simulink model "S_ELECTRO_2025_MTET_NoInt_EnvDatos_V1"  (R2017a)
settings: Solver=FixedStepDiscrete  StartTime=0.0  StopTime=10.0  RelTol=1e-3
undefined symbols (not defined in the file or in its folder): Down, GPTRIP1SEL, GPTRIP2SEL, TZ1, TZ2, Up
libraries: c2802xlib x4, c2806xlib x2, simulink x1, c280xlib x1
settings Model: ExtModeTrigDuration=8  Creator=dricl  LastModifiedBy=dricl
settings OptimizationCC: DefaultUnderspecifiedDataType=single  PassReuseOutputArgsAs=Individual arguments  MaxStackSize=512
settings DebuggingCC: ParameterTunabilityLossMsg=error
settings HardwareCC: ProdBitPerChar=16  ProdBitPerInt=16  ProdBitPerPointer=32  ProdBitPerSizeT=32  ProdBitPerPtrDiffT=32  ProdLargestAtomicInteger=Integer  ProdLargestAtomicFloat=None  ProdWordSize=16  ProdLongLongMode=on  ProdHWDeviceType=Texas Instruments->C2000
settings SFSimCC: MATLABDynamicMemAlloc=off
settings RTWCC: SystemTargetFile=ert.tlc  HardwareBoard=TI Piccolo F2806x  TLCOptions=-aInlineSetEventsForThisBaseRateFcn=TLC_FALSE -aSuppressMultiTaskScheduler=TLC_FALSE -aRateBasedStepFcn=1  TemplateMakefile=ert_default_tmf  Description=Embedded Coder  Toolchain=Texas Instruments Code Composer Studio v5 (C2000)  CodeExecutionProfiling=on  CodeProfilingSaveOptions=AllData  CodeProfilingInstrumentation=on
settings CodeAppCC: ForceParamTrailComments=on  IgnoreCustomStorageClasses=off  OperatorAnnotations=on  SimulinkDataObjDesc=on  SFDataObjDesc=on  MATLABFcnDesc=on  InsertBlockDesc=on  MATLABSourceComments=on
settings ERTTargetCC: CodeReplacementLibrary=TI C28x  MemSecPackage=tic2000demospkg  MemSecFuncExecute=code_ramfuncs

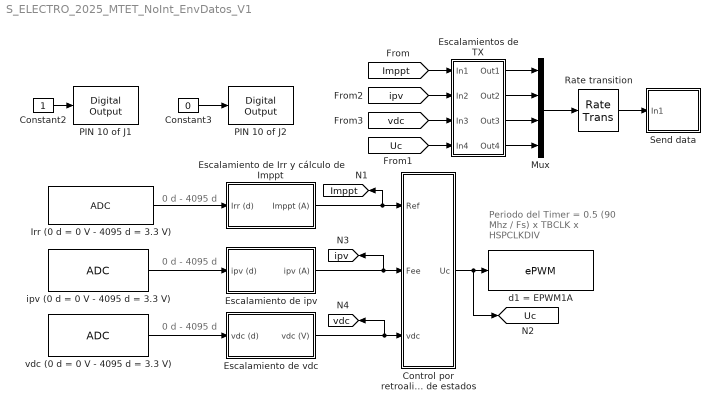
== system S_ELECTRO_2025_MTET_NoInt_EnvDatos_V1 ==
  note: 0 d - 4095 d
  note: Periodo del Timer =
      |  0.5 (90 Mhz / Fs)  x
      | TBCLK x HSPCLKDIV
  note: 0 d - 4095 d
  note: 0 d - 4095 d
  Constant2 : Constant  Priority=1  SampleTime=0.0002
  Constant3 : Constant  Priority=11  Value=0  SampleTime=0.0002
  Control por retroalimentación de estados : Subsystem  Priority=9  TreatAsAtomicUnit=on
  Escalamiento de Irr y cálculo de Imppt : Subsystem  Priority=6  TreatAsAtomicUnit=on
  Escalamiento de ipv : Subsystem  Priority=7  TreatAsAtomicUnit=on
  Escalamiento de vdc : Subsystem  Priority=8  TreatAsAtomicUnit=on
  Escalamientos de TX : Subsystem  TreatAsAtomicUnit=on
  "Irr (0 d = 0 V - 4095 d = 3.3 V) " : c2802xlib/ADC  Priority=3  ADCModule=1  samplingMode=Single sample mode  ADCResolution=12-bit (Single-ended input)  useSOC1=SOC1  useSOC2=SOC0_SOC1  SOCAcquisitionWindow=7  SOCTriggerSource=ePWM1_ADCSOCA  SOCInterruptTrigger=No ADCINT  Ts=0.0002  dType=uint16  postInterrupt=off  interruptSel=ADCINT1  ADCINTContinuous=on  endma=off  chdma=1  blkParamProc=C2000  conv1=ADCINA1  conv2=ADCINA0 and ADCINB0  conv1_Type4=ADCIN0  conv2_Type4=ADCIN0 and ADCIN1
      settings: SourceProductName=Embedded Coder Support Package for Texas Instruments C2000 Processors
  Mux : Mux
  PIN 10 of J1 : c2806xlib/Digital Output  Priority=2  GPIO_Number=GPIO32~GPIO39  GPIO_Bit0=on  GPIO_BIT0_Toggle=off  GPIO_Bit1=off  GPIO_BIT1_Toggle=off  GPIO_Bit2=off  GPIO_BIT2_Toggle=off  GPIO_Bit3=off  GPIO_BIT3_Toggle=off  GPIO_Bit4=off  GPIO_BIT4_Toggle=off  GPIO_Bit5=off  GPIO_BIT5_Toggle=off  GPIO_Bit6=off  GPIO_BIT6_Toggle=off  GPIO_Bit7=off  GPIO_BIT7_Toggle=off
      settings: SourceProductName=Embedded Coder Support Package for Texas Instruments C2000 Processors  SourceProductBaseCode=TIC2000
  PIN 10 of J2 : c2806xlib/Digital Output  Priority=12  GPIO_Number=GPIO32~GPIO39  GPIO_Bit0=on  GPIO_BIT0_Toggle=off  GPIO_Bit1=off  GPIO_BIT1_Toggle=off  GPIO_Bit2=off  GPIO_BIT2_Toggle=off  GPIO_Bit3=off  GPIO_BIT3_Toggle=off  GPIO_Bit4=off  GPIO_BIT4_Toggle=off  GPIO_Bit5=off  GPIO_BIT5_Toggle=off  GPIO_Bit6=off  GPIO_BIT6_Toggle=off  GPIO_Bit7=off  GPIO_BIT7_Toggle=off
      settings: SourceProductName=Embedded Coder Support Package for Texas Instruments C2000 Processors  SourceProductBaseCode=TIC2000
  Rate transition : RateTransition  Integrity=off  Deterministic=off  OutPortSampleTime=0.0002
  Send data : Subsystem  TreatAsAtomicUnit=on
  d1 = EPWM1A : c2802xlib/ePWM  Priority=10  useModule=ePWM1  ePWMxLINKTBPRD=Not Linked  periodUnits=Clock cycles  timerSource=Specify via dialog  timerPeriod_clk=9000  timerPeriod_sec=0.0001  tbshadow=Counter equals to zero  countingMode=Up-Down  phaseActiveEnable=Disable  phaseDirection=Count down after sync  phaseActive=0  synchronizationEnable=off  dcaevt1Sync=off  dcbevt1Sync=off  synchronizationOption=Disable  clockPrescale=1  HSclockPrescale=1  enswap=off  ePWMxAStatus=on  ePWMxAactionLogic1=Do nothing  ePWMxAactionLogic2=Do nothing  ePWMxAactionLogic3=Clear  ePWMxAactionLogic4=Set  ePWMxAactionLogic5=Do nothing  ePWMxAactionLogic6=Do nothing  ePWMxALoadMode=Load on counter equals to zero (CTR=Zero)  ePWMxACSFenable=off  ePWMxACSFvalue=Forcing disable  ePWMxASFreload=Zero  ePWMxBStatus=off  ePWMxBactionLogic1=Set  ePWMxBactionLogic2=Clear  ePWMxBactionLogic3=Do nothing  ePWMxBactionLogic4=Do nothing  ePWMxBactionLogic5=Clear  ePWMxBactionLogic6=Set  ePWMxBLoadMode=Load on counter equals to zero (CTR=Zero)  ePWMxBCSFenable=off  ePWMxBCSFvalue=Forcing disable  ePWMxBSFreload=Zero  ePWNxBOutWay=off  ePWMxLINKCMPA=Not Linked  CMPAUnits=Clock cycles  CMPASource=Input port  CMPAValue_per=50  CMPAValue_clk=4500  enCMPAshadow=Counter equals to zero  ePWMxLINKCMPB=Not Linked  CMPBUnits=Clock cycles  CMPBSource=Specify via dialog  CMPBValue_per=50  CMPBValue_clk=4500  enCMPBshadow=Counter equals to zero  ePWMxLINKCMPC=Not Linked  CMPCUnits=Clock cycles  CMPCSource=Specify via dialog  CMPCValue_per=50  CMPCValue_clk=32000  enCMPCshadow=Counter equals to zero  ePWMxLINKCMPD=Not Linked  CMPDUnits=Clock cycles  CMPDSource=Specify via dialog  CMPDValue_per=50  CMPDValue_clk=32000  enCMPDshadow=Counter equals to zero  enableDBePWMxA=on  enableDBePWMxB=on  enhalfcycle=off  DBpolarity=Active high complementary (AHC)  DBedgeDelay=Positive  DBSource_ePWMxA=ePWMxA  DBSource_ePWMxB=ePWMxA  DBperiodSource=Specify via dialog  REDperiod=50  FEDperiod=50  adcstartModuleA=on  adcrequestEventA=First event  adcstartEventA=Counter equals to period (CTR=PRD)  adcstartEventA_type2=Digital Compare Module A Event 1 start of conversion (DCAEVT1.soc)  adcstartModuleB=off  adcrequestEventB=First event  adcstartEventB=Counter equals to zero (CTR=Zero)  adcstartEventB_type2=Counter equals to zero (CTR=Zero)  intEn=off  intPrd=First event  intSel=Counter equals to zero (CTR=Zero)  intSel_type2=Counter equals to zero (CTR=Zero)  hrpe=off  enHRPWM=off  HRPWM_LoadMode=Counter equals to period (CTR=PRD)  HRPWM_CTLMode=Duty or Period control mode  HRPWM_EDGMode=Both edge  hrpeb=off  enHRPWMB=off  HRPWM_LoadModeB=Counter equals to zero (CTR=ZERO)  HRPWM_CTLModeB=Duty or Period control mode  HRPWM_EDGModeB=Both edge  enSFO=on  enautoconv=on  chopperEnable=off  chopperFrequency=1  chopperFirstwidth=1  chopperDuty=12.5%  tripZonesource=Specify via dialog  tzselOSHT1=off  tzselOSHT2=off  tzselOSHT3=off  tzselOSHDCAEV1=off  tzselOSHDCBEV1=off  tzselCBC1=off  tzselCBC2=off  tzselCBC3=off  tzselCBCDCAEV2=off  tzselCBCDCBEV2=off  tzselOSHT4=off  tzselOSHT5=off  tzselOSHT6=off  tzselCBC4=off  tzselCBC5=off  tzselCBC6=off  enTzOstIntr=off  enTzCbcIntr=off  enTzDCAEVT1Intr=off  enTzDCAEVT2Intr=off  enTzDCBEVT1Intr=off  enTzDCBEVT2Intr=off  ePWMxAforced=No action  ePWMxBforced=No action  DCAEVT1forced=No action  DCBEVT1forced=No action  DCAEVT2forced=No action  DCBEVT2forced=No action  dcah=Trip Zone 1 input (TZ1)  dcal=Trip Zone 2 input (TZ2)  dcbh=Trip Zone 1 input (TZ1)  dcbl=Trip Zone 2 input (TZ2)  dcah_type2=GPTRIP1SEL/(TZ1)  dcal_type2=GPTRIP2SEL/(TZ2)  dcbh_type2=GPTRIP1SEL/(TZ1)  dcbl_type2=GPTRIP2SEL/(TZ2)  gendcaevt1=Event disabled  gendcaevt2=Event disabled  gendcbevt1=Event disabled  gendcbevt2=Event disabled  dcaevt1src=DCAEVT1 with sync  dcaevt2src=DCAEVT2 with sync  dcbevt1src=DCBEVT1 with sync  dcbevt2src=DCBEVT2 with sync  pulsesel=Counter equals to zero (CTR=Zero)  blankinv=off  blankoffset=0  blankwidth=0  evsrcsel=Filtered version of DCAEVT1 (DCAEVT1FILT)  encape=off  PwmType=C2000
      settings: SourceProductName=Embedded Coder Support Package for Texas Instruments C2000 Processors
  "ipv (0 d = 0 V - 4095 d = 3.3 V) " : c2802xlib/ADC  Priority=4  ADCModule=1  samplingMode=Single sample mode  ADCResolution=12-bit (Single-ended input)  useSOC1=SOC2  useSOC2=SOC0_SOC1  SOCAcquisitionWindow=7  SOCTriggerSource=ePWM1_ADCSOCA  SOCInterruptTrigger=No ADCINT  Ts=0.0002  dType=uint16  postInterrupt=off  interruptSel=ADCINT1  ADCINTContinuous=on  endma=off  chdma=1  blkParamProc=C2000  conv1=ADCINA0  conv2=ADCINA0 and ADCINB0  conv1_Type4=ADCIN0  conv2_Type4=ADCIN0 and ADCIN1
      settings: SourceProductName=Embedded Coder Support Package for Texas Instruments C2000 Processors
  "vdc (0 d = 0 V - 4095 d = 3.3 V) " : c2802xlib/ADC  Priority=5  ADCModule=1  samplingMode=Single sample mode  ADCResolution=12-bit (Single-ended input)  useSOC1=SOC3  useSOC2=SOC0_SOC1  SOCAcquisitionWindow=7  SOCTriggerSource=ePWM1_ADCSOCA  SOCInterruptTrigger=No ADCINT  Ts=0.0002  dType=uint16  postInterrupt=off  interruptSel=ADCINT1  ADCINTContinuous=on  endma=off  chdma=1  blkParamProc=C2000  conv1=ADCINA2  conv2=ADCINA0 and ADCINB0  conv1_Type4=ADCIN0  conv2_Type4=ADCIN0 and ADCIN1
      settings: SourceProductName=Embedded Coder Support Package for Texas Instruments C2000 Processors
  tag scope: Imppt=global, Uc=global, ipv=global, vdc=global
  wires:
  Escalamiento de ipv/1(ipv (A)) -> [ipv], Control por retroalimentación de estados/2(Fee)
  "ipv (0 d = 0 V - 4095 d = 3.3 V) "/1 -> Escalamiento de ipv/1(ipv (d))
  Escalamiento de Irr y cálculo de Imppt/1(Imppt (A)) -> [Imppt], Control por retroalimentación de estados/1(Ref)
  "Irr (0 d = 0 V - 4095 d = 3.3 V) "/1 -> Escalamiento de Irr y cálculo de Imppt/1(Irr (d))
  Constant2/1 -> PIN 10 of J1/1
  Constant3/1 -> PIN 10 of J2/1
  "vdc (0 d = 0 V - 4095 d = 3.3 V) "/1 -> Escalamiento de vdc/1(vdc (d))
  Escalamiento de vdc/1(vdc (V)) -> [vdc], Control por retroalimentación de estados/3(vdc)
  [vdc] -> Escalamientos de TX/3(In3)
  [ipv] -> Escalamientos de TX/2(In2)
  [Uc] -> Escalamientos de TX/4(In4)
  [Imppt] -> Escalamientos de TX/1(In1)
  Escalamientos de TX/2(Out2) -> Mux/2
  Escalamientos de TX/4(Out4) -> Mux/4
  Escalamientos de TX/3(Out3) -> Mux/3
  Escalamientos de TX/1(Out1) -> Mux/1
  Mux/1 -> Rate transition/1
  Rate transition/1 -> Send data/1(In1)
  Control por retroalimentación de estados/1(Uc) -> [Uc], d1 = EPWM1A/1

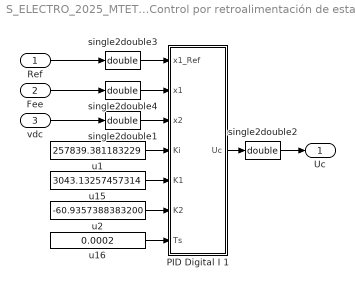
== system S_ELECTRO_2025_MTET_NoInt_EnvDatos_V1/Control por retroalimentación de estados ==
  Ref : Inport
  Fee : Inport  Port=2
  vdc : Inport  Port=3
  PID Digital I 1 : MATLAB Function  TreatAsAtomicUnit=on
  single2double{1..4} (4 alike) : DataTypeConversion  OutDataTypeStr=double
  u1 : Constant  Value=257839.381183229  SampleTime=0.0002
  u15 : Constant  Value=3043.13257457314  SampleTime=0.0002
  u16 : Constant  Value=0.0002  SampleTime=0.0002
  u2 : Constant  Value=-60.9357388383200  SampleTime=0.0002
  Uc : Outport
  wires:
  u16/1 -> PID Digital I 1/7(Ts)
  Ref/1 -> single2double3/1
  single2double2/1 -> Uc/1
  Fee/1 -> single2double4/1
  PID Digital I 1/1(Uc) -> single2double2/1
  single2double3/1 -> PID Digital I 1/1(x1_Ref)
  single2double4/1 -> PID Digital I 1/2(x1)
  u1/1 -> PID Digital I 1/4(Ki)
  vdc/1 -> single2double1/1
  single2double1/1 -> PID Digital I 1/3(x2)
  u15/1 -> PID Digital I 1/5(K1)
  u2/1 -> PID Digital I 1/6(K2)

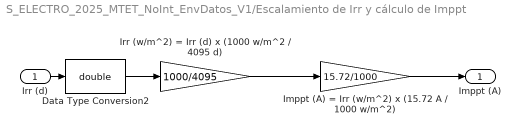
== system S_ELECTRO_2025_MTET_NoInt_EnvDatos_V1/Escalamiento de Irr y cálculo de Imppt ==
  Irr (d) : Inport
  Data Type Conversion2 : DataTypeConversion  OutDataTypeStr=double
  "Imppt (A) = Irr (w/m^2) x (15.72 A / 1000 w/m^2) " : Gain  Gain=15.72/1000
  Irr (w/m^2) = Irr (d) x (1000 w/m^2 / 4095 d) : Gain  Gain=1000/4095
  Imppt (A) : Outport
  wires:
  Irr (d)/1 -> Data Type Conversion2/1
  Data Type Conversion2/1 -> Irr (w/m^2) = Irr (d) x (1000 w/m^2 / 4095 d)/1
  Irr (w/m^2) = Irr (d) x (1000 w/m^2 / 4095 d)/1 -> "Imppt (A) = Irr (w/m^2) x (15.72 A / 1000 w/m^2) "/1
  "Imppt (A) = Irr (w/m^2) x (15.72 A / 1000 w/m^2) "/1 -> Imppt (A)/1

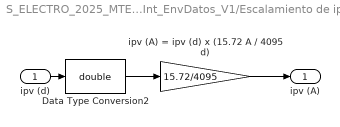
== system S_ELECTRO_2025_MTET_NoInt_EnvDatos_V1/Escalamiento de ipv ==
  ipv (d) : Inport
  Data Type Conversion2 : DataTypeConversion  OutDataTypeStr=double
  ipv (A) = ipv (d) x (15.72 A / 4095 d) : Gain  Gain=15.72/4095
  ipv (A) : Outport
  wires:
  ipv (d)/1 -> Data Type Conversion2/1
  Data Type Conversion2/1 -> ipv (A) = ipv (d) x (15.72 A / 4095 d)/1
  ipv (A) = ipv (d) x (15.72 A / 4095 d)/1 -> ipv (A)/1

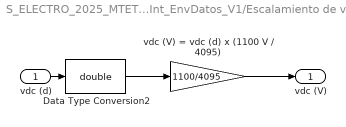
== system S_ELECTRO_2025_MTET_NoInt_EnvDatos_V1/Escalamiento de vdc ==
  vdc (d) : Inport
  Data Type Conversion2 : DataTypeConversion  OutDataTypeStr=double
  vdc (V) = vdc (d) x (1100 V / 4095) : Gain  Gain=1100/4095
  vdc (V) : Outport
  wires:
  Data Type Conversion2/1 -> vdc (V) = vdc (d) x (1100 V / 4095)/1
  vdc (d)/1 -> Data Type Conversion2/1
  vdc (V) = vdc (d) x (1100 V / 4095)/1 -> vdc (V)/1

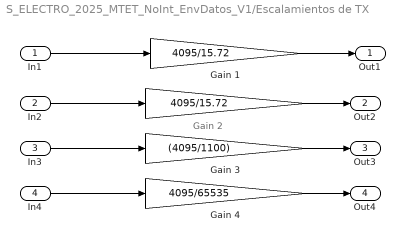
== system S_ELECTRO_2025_MTET_NoInt_EnvDatos_V1/Escalamientos de TX ==
  note: Gain 2
  In1 : Inport
  In2 : Inport  Port=2
  In3 : Inport  Port=3
  In4 : Inport  Port=4
  " " : Gain  Gain=4095/15.72  OutDataTypeStr=uint16  RndMeth=Simplest
  Gain 1 : Gain  Gain=4095/15.72  OutDataTypeStr=uint16  RndMeth=Simplest
  Gain 3 : Gain  Gain=(4095/1100)  OutDataTypeStr=uint16  RndMeth=Simplest
  Gain 4 : Gain  Gain=4095/65535  OutDataTypeStr=uint16  RndMeth=Simplest
  Out1 : Outport
  Out2 : Outport  Port=2
  Out3 : Outport  Port=3
  Out4 : Outport  Port=4
  wires:
  Gain 1/1 -> Out1/1
  " "/1 -> Out2/1
  Gain 3/1 -> Out3/1
  In1/1 -> Gain 1/1
  In2/1 -> " "/1
  In3/1 -> Gain 3/1
  In4/1 -> Gain 4/1
  Gain 4/1 -> Out4/1

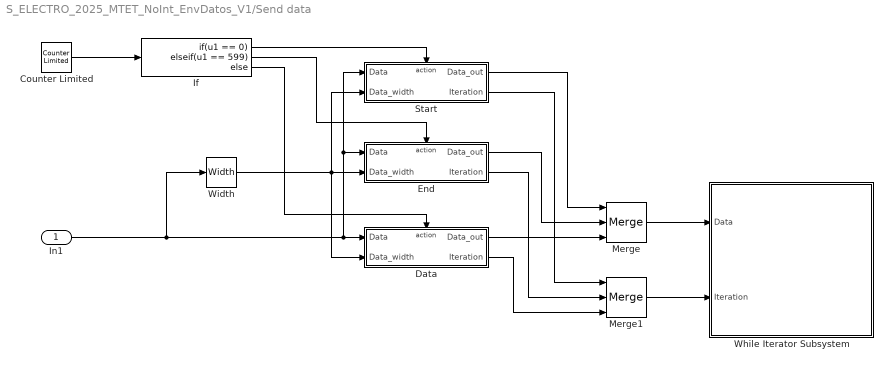
== system S_ELECTRO_2025_MTET_NoInt_EnvDatos_V1/Send data ==
  In1 : Inport
  Counter Limited : simulink/Sources/Counter Limited  uplimit=599  tsamp=-1
  Data : Subsystem  TreatAsAtomicUnit=on
  End : Subsystem  TreatAsAtomicUnit=on
  If : If  IfExpression=u1 == 0  ElseIfExpressions=u1 == 599
  Merge : Merge  Inputs=3
  Merge1 : Merge  Inputs=3
  Start : Subsystem  TreatAsAtomicUnit=on
  While Iterator Subsystem : Subsystem  TreatAsAtomicUnit=on
  Width : Width  OutDataTypeMode=All ports same datatype  DataType=uint16
  wires:
  If/1 -> Start/Action
  If/2 -> End/Action
  If/3 -> Data/Action
  Counter Limited/1 -> If/1
  Start/1(Data_out) -> Merge/1
  End/1(Data_out) -> Merge/2
  Data/1(Data_out) -> Merge/3
  Merge/1 -> While Iterator Subsystem/1(Data)
  Merge1/1 -> While Iterator Subsystem/2(Iteration)
  Start/2(Iteration) -> Merge1/1
  End/2(Iteration) -> Merge1/2
  Data/2(Iteration) -> Merge1/3
  In1/1 -> Width/1, Start/1(Data), End/1(Data), Data/1(Data)
  Width/1 -> Data/2(Data_width), Start/2(Data_width), End/2(Data_width)

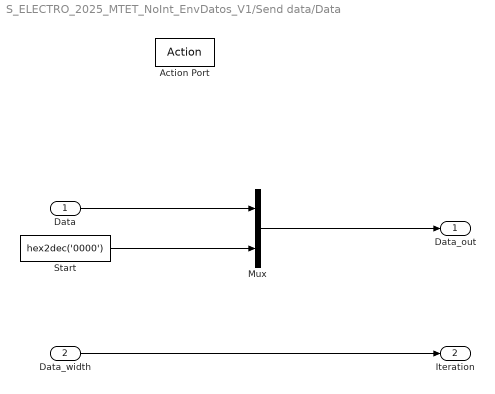
== system S_ELECTRO_2025_MTET_NoInt_EnvDatos_V1/Send data/Data ==
  Data : Inport
  Data_width : Inport  Port=2
  Action Port : ActionPort  ActionType=else
  Mux : Mux  Inputs=2
  Start : Constant  Value=hex2dec('0000')  OutDataTypeStr=uint16
  Data_out : Outport
  Iteration : Outport  Port=2
  wires:
  Start/1 -> Mux/2
  Mux/1 -> Data_out/1
  Data/1 -> Mux/1
  Data_width/1 -> Iteration/1

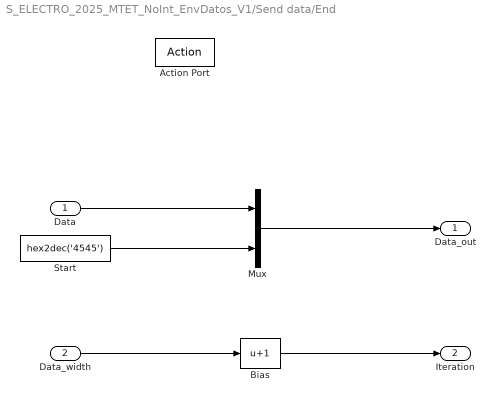
== system S_ELECTRO_2025_MTET_NoInt_EnvDatos_V1/Send data/End ==
  Data : Inport
  Data_width : Inport  Port=2
  Action Port : ActionPort  ActionType=elseif
  Bias : Bias  Bias=1
  Mux : Mux  Inputs=2
  Start : Constant  Value=hex2dec('4545')  OutDataTypeStr=uint16
  Data_out : Outport
  Iteration : Outport  Port=2
  wires:
  Mux/1 -> Data_out/1
  Data_width/1 -> Bias/1
  Start/1 -> Mux/2
  Bias/1 -> Iteration/1
  Data/1 -> Mux/1

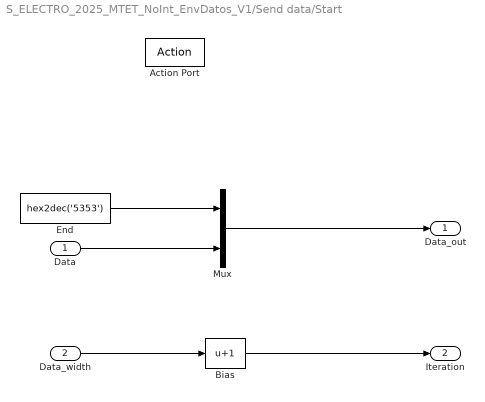
== system S_ELECTRO_2025_MTET_NoInt_EnvDatos_V1/Send data/Start ==
  Data : Inport
  Data_width : Inport  Port=2
  Action Port : ActionPort  ActionType=then
  Bias : Bias  Bias=1
  End : Constant  Value=hex2dec('5353')  OutDataTypeStr=uint16
  Mux : Mux  Inputs=2
  Data_out : Outport
  Iteration : Outport  Port=2
  wires:
  End/1 -> Mux/1
  Mux/1 -> Data_out/1
  Data_width/1 -> Bias/1
  Bias/1 -> Iteration/1
  Data/1 -> Mux/2

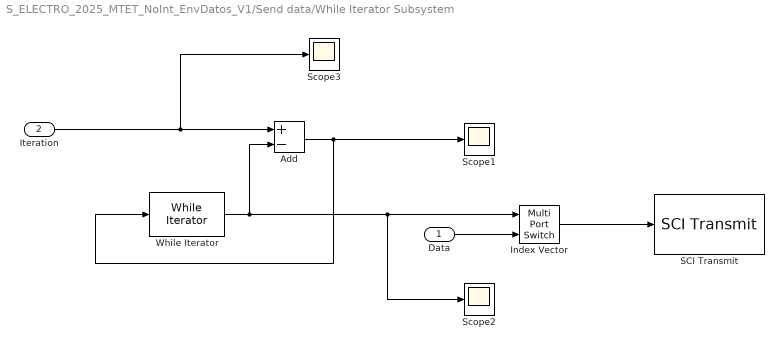
== system S_ELECTRO_2025_MTET_NoInt_EnvDatos_V1/Send data/While Iterator Subsystem ==
  Data : Inport
  Iteration : Inport  Port=2
  Add : Sum  Inputs=+-  OutDataTypeStr=Inherit: Same as first input
  Index Vector : MultiPortSwitch  Inputs=1
  SCI Transmit : c280xlib/SCI Transmit  sciModule=A  dataHead=''  dataTail=''  postInterrupt=off  numFifo=1
      settings: SourceProductName=Embedded Coder Support Package for Texas Instruments C2000 Processors
  Scope1 : Scope
  Scope2 : Scope
  Scope3 : Scope
  While Iterator : WhileIterator  MaxIters=-1  WhileBlockType=do-while  ShowIterationPort=on  OutputDataType=int16
  wires:
  Iteration/1 -> Scope3/1, Add/1
  Add/1 -> Scope1/1, While Iterator/1
  Index Vector/1 -> SCI Transmit/1
  Data/1 -> Index Vector/2
  While Iterator/1 -> Scope2/1, Index Vector/1, Add/2

== matlab function S_ELECTRO_2025_MTET_NoInt_EnvDatos_V1/Control por retroalimentación de estados/PID Digital I 1 ==
  data: x1_Ref input; x1 input; x2 input; Uc output; Ki input; K1 input; K2 input; Ts input
function Uc = fcn(x1_Ref, x1, x2, Ki, K1, K2, Ts)
    % Retroalimentación de estados con acción integral
    
    % Variables persistentes para mantener el estado entre llamadas
    persistent ek Acc_Int Acc_Int_1 uk
    
    if isempty(ek)
        ek = 0;
        Acc_Int = 0;
        Acc_Int_1 = 0;
        uk = 0;
    end

    % Cálculo del error
    ek = x1_Ref - x1;

    % Acción integral
    Acc_Int = Ki * ek * Ts + Acc_Int_1;
    Acc_Int_1 = Acc_Int;

    % Ley de control: acción integral menos retroalimentación de estados
    uk = Acc_Int - (K1 * x1 + K2 * x2);

    % Saturación (opcional)
    %uk = min(max(uk, 0), 65535); %Para med TET
     uk = min(max(uk, 0), 9000);  %Para pruebas de TX/RX 

    % Salida del controlador
    Uc = uk;
end
